simulink model "raMPTEEST"  (R2012b)
settings: Solver=FixedStepDiscrete  StartTime=0.0  StopTime=10.0  RelTol=1e-3
libraries: c28xdmclib x1, idelinklib_tgtpref x1
settings Model: Creator=Krunal  LastModifiedBy=Krunal
settings DataIOCC: SaveOutput=off  SaveTime=off
settings OptimizationCC: OptimizeModelRefInitCode=on  LifeSpan=1
settings HardwareCC: ProdBitPerChar=16  ProdBitPerInt=16  ProdBitPerPointer=16  ProdLargestAtomicInteger=Integer  ProdIntDivRoundTo=Zero  ProdEndianess=LittleEndian  ProdWordSize=16  ProdHWDeviceType=Texas Instruments->C2000  TargetBitPerChar=16  TargetBitPerInt=16  TargetBitPerPointer=16  TargetLargestAtomicInteger=Integer  TargetIntDivRoundTo=Zero  TargetEndianess=LittleEndian  TargetWordSize=16  TargetHWDeviceType=Texas Instruments->C2000  ProdEqTarget=off
settings RTWCC: SystemTargetFile=idelink_ert.tlc  GenerateMakefile=off  TemplateMakefile=none  Description=IDE Link ERT  ProcessScript=idelink_ert_make_rtw_hook
settings CodeAppCC: IgnoreCustomStorageClasses=off

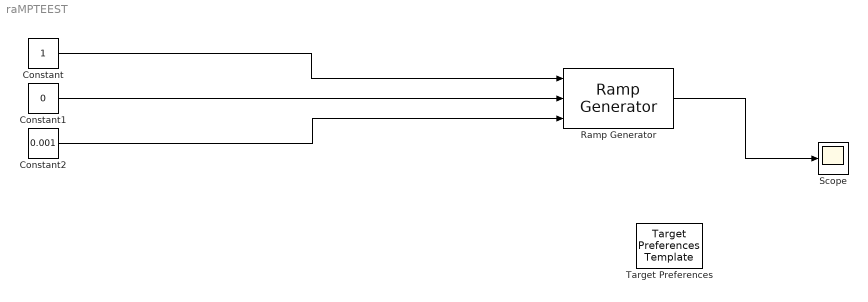
== system raMPTEEST ==
  Constant : Constant  OutDataTypeStr=fixdt(1,32,2^-9,0)  SampleTime=0.001
  Constant1 : Constant  Value=0  OutDataTypeStr=fixdt(1,32,2^-9,0)
  Constant2 : Constant  Value=0.001  OutDataTypeStr=fixdt(1,32,2^-9,0)
  Ramp Generator : c28xdmclib/Ramp Generator  step_angle_max=1
  Scope : Scope
  Target Preferences : idelinklib_tgtpref/Target Preferences Template  Tag=ccslinktgtpref_ccsv5  library=off
  wires:
  Ramp Generator/1 -> Scope/1
  Constant2/1 -> Ramp Generator/3
  Constant1/1 -> Ramp Generator/2
  Constant/1 -> Ramp Generator/1
